simulink model "pv_array"  (Simulink 10.0)
settings: Solver=ode45  StartTime=0.0  StopTime=1.0  RelTol=1e-3  EnableMultiTasking=on
libraries: simulink x8
settings Model: Creator=motahhir  LastModifiedBy=bhisma
settings DataIOCC: LimitDataPoints=on  SignalLoggingSaveFormat=ModelDataLogs
settings OptimizationCC: ExpressionDepthLimit=2147483647
settings DebuggingCC: SolverPrmCheckMsg=warning  FcnCallInpInsideContextMsg=warning  StateNameClashWarn=warning  SFExecutionAtInitializationDiag=warning
settings GRTTargetCC: GeneratePreprocessorConditionals=Disable all  CombineOutputUpdateFcns=on  GRTInterface=off
settings ConfigComp: CovExternalEMLEnable=off  CovSFcnEnable=off

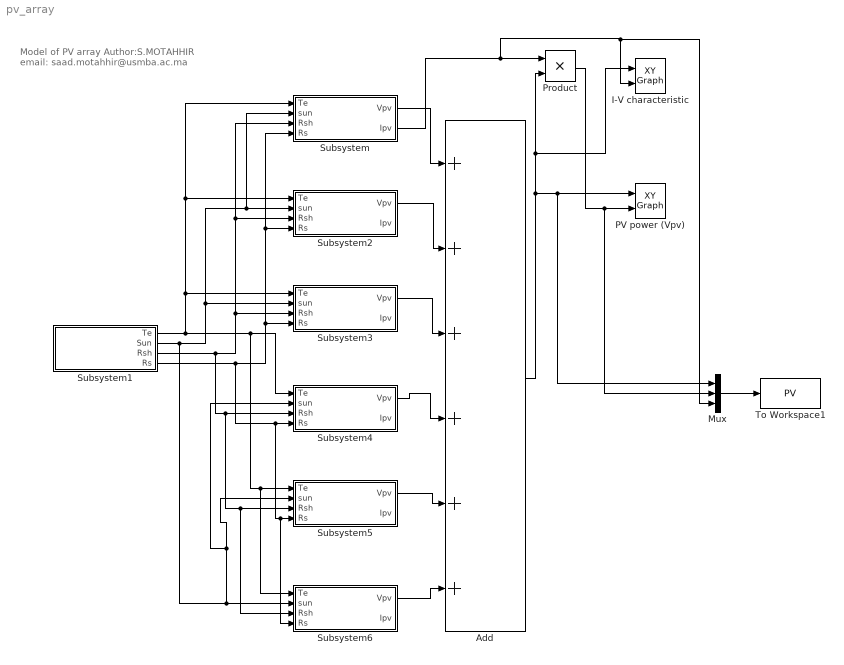
== system pv_array ==
  note: Model of PV array
      | Author:S.MOTAHHIR
      | email: saad.motahhir@usmba.ac.ma
  Add : Sum  Inputs=++++++
  I-V characteristic : simulink/Sinks/XY Graph  xmin=0  xmax=130  ymin=0  ymax=4  st=-1
  Mux : Mux  Inputs=3
  PV power (Vpv) : simulink/Sinks/XY Graph  xmin=0  xmax=130  ymin=0  ymax=400  st=-1
  Product : Product  RndMeth=Zero
  Subsystem : Subsystem
      mask Display:
      | plot([0.3 0.4],[0.4 0.8]);
      | plot([0.4 0.5],[0.4 0.8]);
      | plot([0.5 0.6],[0.4 0.8]);
      | plot([0.6 0.7],[0.4 0.8]);
      | plot([0.3 0.6],[0.4 0.4]);
      | plot([0.325 0.625],[0.5 0.5]);
      | plot([0.35 0.65],[0.6 0.6]);
      | plot([0.375 0.675],[0.7 0.7]);
      | plot([0.4 0.7],[0.8 0.8]);
      | text(0.5,0.9,'PV module (V)','horizontalAlignment', 'center');
  Subsystem1 : Subsystem
  Subsystem2 : Subsystem
      mask Display:
      | plot([0.3 0.4],[0.4 0.8]);
      | plot([0.4 0.5],[0.4 0.8]);
      | plot([0.5 0.6],[0.4 0.8]);
      | plot([0.6 0.7],[0.4 0.8]);
      | plot([0.3 0.6],[0.4 0.4]);
      | plot([0.325 0.625],[0.5 0.5]);
      | plot([0.35 0.65],[0.6 0.6]);
      | plot([0.375 0.675],[0.7 0.7]);
      | plot([0.4 0.7],[0.8 0.8]);
      | text(0.5,0.9,'PV module (V)','horizontalAlignment', 'center');
  Subsystem3 : Subsystem
      mask Display:
      | plot([0.3 0.4],[0.4 0.8]);
      | plot([0.4 0.5],[0.4 0.8]);
      | plot([0.5 0.6],[0.4 0.8]);
      | plot([0.6 0.7],[0.4 0.8]);
      | plot([0.3 0.6],[0.4 0.4]);
      | plot([0.325 0.625],[0.5 0.5]);
      | plot([0.35 0.65],[0.6 0.6]);
      | plot([0.375 0.675],[0.7 0.7]);
      | plot([0.4 0.7],[0.8 0.8]);
      | text(0.5,0.9,'PV module (V)','horizontalAlignment', 'center');
  Subsystem4 : Subsystem
      mask Display:
      | plot([0.3 0.4],[0.4 0.8]);
      | plot([0.4 0.5],[0.4 0.8]);
      | plot([0.5 0.6],[0.4 0.8]);
      | plot([0.6 0.7],[0.4 0.8]);
      | plot([0.3 0.6],[0.4 0.4]);
      | plot([0.325 0.625],[0.5 0.5]);
      | plot([0.35 0.65],[0.6 0.6]);
      | plot([0.375 0.675],[0.7 0.7]);
      | plot([0.4 0.7],[0.8 0.8]);
      | text(0.5,0.9,'PV module (V)','horizontalAlignment', 'center');
  Subsystem5 : Subsystem
      mask Display:
      | plot([0.3 0.4],[0.4 0.8]);
      | plot([0.4 0.5],[0.4 0.8]);
      | plot([0.5 0.6],[0.4 0.8]);
      | plot([0.6 0.7],[0.4 0.8]);
      | plot([0.3 0.6],[0.4 0.4]);
      | plot([0.325 0.625],[0.5 0.5]);
      | plot([0.35 0.65],[0.6 0.6]);
      | plot([0.375 0.675],[0.7 0.7]);
      | plot([0.4 0.7],[0.8 0.8]);
      | text(0.5,0.9,'PV module (V)','horizontalAlignment', 'center');
  Subsystem6 : Subsystem
      mask Display:
      | plot([0.3 0.4],[0.4 0.8]);
      | plot([0.4 0.5],[0.4 0.8]);
      | plot([0.5 0.6],[0.4 0.8]);
      | plot([0.6 0.7],[0.4 0.8]);
      | plot([0.3 0.6],[0.4 0.4]);
      | plot([0.325 0.625],[0.5 0.5]);
      | plot([0.35 0.65],[0.6 0.6]);
      | plot([0.375 0.675],[0.7 0.7]);
      | plot([0.4 0.7],[0.8 0.8]);
      | text(0.5,0.9,'PV module (V)','horizontalAlignment', 'center');
  To Workspace1 : ToWorkspace  VariableName=PV  SaveFormat=Structure With Time  SampleTime=-1
  wires:
  Subsystem1/1(Te) -> Subsystem3/1(Te), Subsystem2/1(Te), Subsystem/1(Te), Subsystem4/1(Te), Subsystem6/1(Te), Subsystem5/1(Te)
  Subsystem1/3(Rsh) -> Subsystem3/3(Rsh), Subsystem2/3(Rsh), Subsystem/3(Rsh), Subsystem4/3(Rsh), Subsystem6/3(Rsh), Subsystem5/3(Rsh)
  Subsystem1/4(Rs) -> Subsystem3/4(Rs), Subsystem2/4(Rs), Subsystem/4(Rs), Subsystem4/4(Rs), Subsystem6/4(Rs), Subsystem5/4(Rs)
  Subsystem/1(Vpv) -> Add/1
  Subsystem2/1(Vpv) -> Add/2
  Subsystem3/1(Vpv) -> Add/3
  Subsystem4/1(Vpv) -> Add/4
  Subsystem5/1(Vpv) -> Add/5
  Subsystem6/1(Vpv) -> Add/6
  Product/1 -> Mux/2, PV power (Vpv)/2
  Mux/1 -> To Workspace1/1
  Add/1 -> Product/2, I-V characteristic/1, Mux/1, PV power (Vpv)/1
  Subsystem/2(Ipv) -> Product/1, Mux/3, I-V characteristic/2
  Subsystem1/2(Sun) -> Subsystem4/2(sun), Subsystem5/2(sun), Subsystem6/2(sun), Subsystem3/2(sun), Subsystem/2(sun), Subsystem2/2(sun)

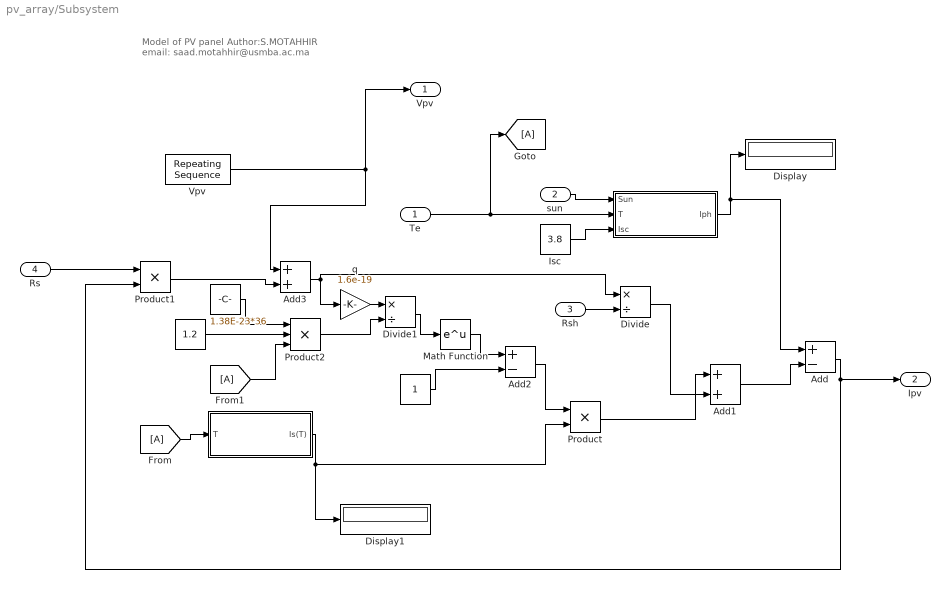
== system pv_array/Subsystem ==
  note: Model of PV panel
      | Author:S.MOTAHHIR
      | email: saad.motahhir@usmba.ac.ma
  Te : Inport
  sun : Inport  Port=2
  Rsh : Inport  Port=3
  Rs : Inport  Port=4
  "  " : Subsystem
  "   " : Subsystem
      mask init:
      | q=1.6e-19;
      | T=298.15;
      | Tnom=298.15;
      | K=1,3806505e-23;
      | N=1.5;
      | vt=36*T*K/q;
      | Is=2.16e-8;
      | Eg=1.12;
  "           " : Constant
  "              " : Constant  Value=1.2
  "               " : Constant  Value=1.38E-23*36
  Add : Sum  Inputs=+-
  Add1 : Sum
  Add2 : Sum  Inputs=+-
  Add3 : Sum
  Display : Display
  Display1 : Display
  Divide : Product  Inputs=*/
  Divide1 : Product  Inputs=*/
  Isc : Constant  Value=3.8
  Math Function : Math  SaturateOnIntegerOverflow=on
  Product : Product  RndMeth=Zero
  Product1 : Product  RndMeth=Zero
  Product2 : Product  Inputs=3  RndMeth=Zero
  "Vpv      " : simulink/Sources/Repeating Sequence  rep_seq_t=[0 1 2]  rep_seq_y="[-0.1  21.5 -0.1]"
  q : Gain  Gain=1.6e-19
  Vpv : Outport
  Ipv : Outport  Port=2
  wires:
  Isc/1 -> "  "/3(Isc)
  Te/1 -> "  "/2(T), [A]
  "  "/1(Iph) -> Display/1, Add/1
  [A] -> "   "/1(T)
  Divide/1 -> Add1/2
  "   "/1(Is(T)) -> Product/2, Display1/1
  Add2/1 -> Product/1
  Math Function/1 -> Add2/1
  "           "/1 -> Add2/2
  Divide1/1 -> Math Function/1
  Product/1 -> Add1/1
  Add1/1 -> Add/2
  q/1 -> Divide1/1
  Add3/1 -> q/1, Divide/1
  "               "/1 -> Product2/1
  [A] -> Product2/3
  "              "/1 -> Product2/2
  Product2/1 -> Divide1/2
  sun/1 -> "  "/1(Sun)
  Rsh/1 -> Divide/2
  Add/1 -> Product1/2, Ipv/1
  Rs/1 -> Product1/1
  Product1/1 -> Add3/2
  "Vpv      "/1 -> Vpv/1, Add3/1

== system pv_array/Subsystem1 ==
  Constant : Constant  Value=298.15
  Constant1 : Constant  Value=1000
  Constant2 : Constant  Value=1000*6
  Constant3 : Constant  Value=0.008*6
  Te : Outport
  Sun : Outport  Port=2
  Rsh : Outport  Port=3
  Rs : Outport  Port=4
  wires:
  Constant/1 -> Te/1
  Constant1/1 -> Sun/1
  Constant3/1 -> Rs/1
  Constant2/1 -> Rsh/1

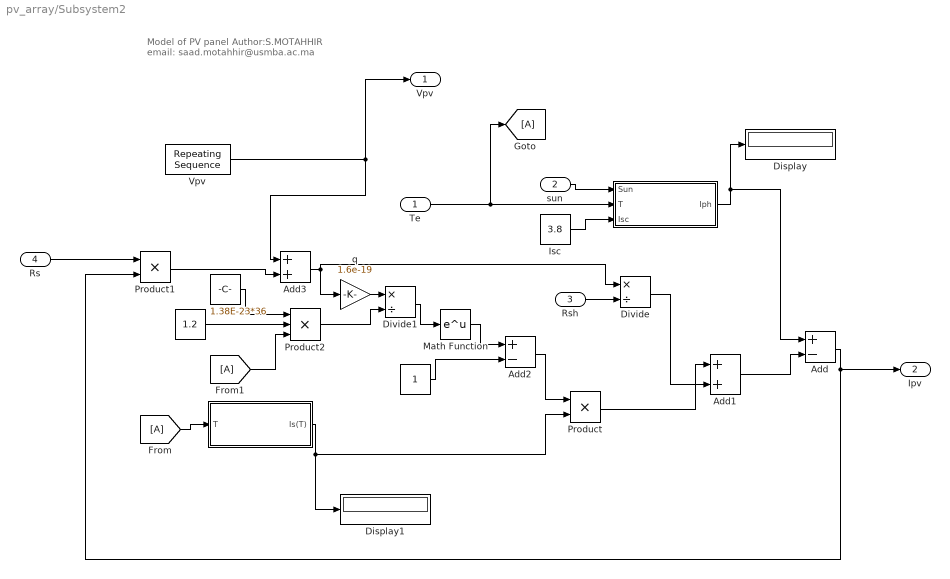
== system pv_array/Subsystem2 ==
  note: Model of PV panel
      | Author:S.MOTAHHIR
      | email: saad.motahhir@usmba.ac.ma
  Te : Inport
  sun : Inport  Port=2
  Rsh : Inport  Port=3
  Rs : Inport  Port=4
  "  " : Subsystem
  "   " : Subsystem
      mask init:
      | q=1.6e-19;
      | T=298.15;
      | Tnom=298.15;
      | K=1,3806505e-23;
      | N=1.5;
      | vt=36*T*K/q;
      | Is=2.16e-8;
      | Eg=1.12;
  "           " : Constant
  "              " : Constant  Value=1.2
  "               " : Constant  Value=1.38E-23*36
  Add : Sum  Inputs=+-
  Add1 : Sum
  Add2 : Sum  Inputs=+-
  Add3 : Sum
  Display : Display
  Display1 : Display
  Divide : Product  Inputs=*/
  Divide1 : Product  Inputs=*/
  Isc : Constant  Value=3.8
  Math Function : Math  SaturateOnIntegerOverflow=on
  Product : Product  RndMeth=Zero
  Product1 : Product  RndMeth=Zero
  Product2 : Product  Inputs=3  RndMeth=Zero
  "Vpv      " : simulink/Sources/Repeating Sequence  rep_seq_t=[0 1 2]  rep_seq_y="[-0.1  21.5 -0.1]"
  q : Gain  Gain=1.6e-19
  Vpv : Outport
  Ipv : Outport  Port=2
  wires:
  Isc/1 -> "  "/3(Isc)
  Te/1 -> "  "/2(T), [A]
  "  "/1(Iph) -> Display/1, Add/1
  [A] -> "   "/1(T)
  Divide/1 -> Add1/2
  "   "/1(Is(T)) -> Product/2, Display1/1
  Add2/1 -> Product/1
  Math Function/1 -> Add2/1
  "           "/1 -> Add2/2
  Divide1/1 -> Math Function/1
  Product/1 -> Add1/1
  Add1/1 -> Add/2
  q/1 -> Divide1/1
  Add3/1 -> q/1, Divide/1
  "               "/1 -> Product2/1
  [A] -> Product2/3
  "              "/1 -> Product2/2
  Product2/1 -> Divide1/2
  sun/1 -> "  "/1(Sun)
  Rsh/1 -> Divide/2
  Add/1 -> Product1/2, Ipv/1
  Rs/1 -> Product1/1
  Product1/1 -> Add3/2
  "Vpv      "/1 -> Vpv/1, Add3/1

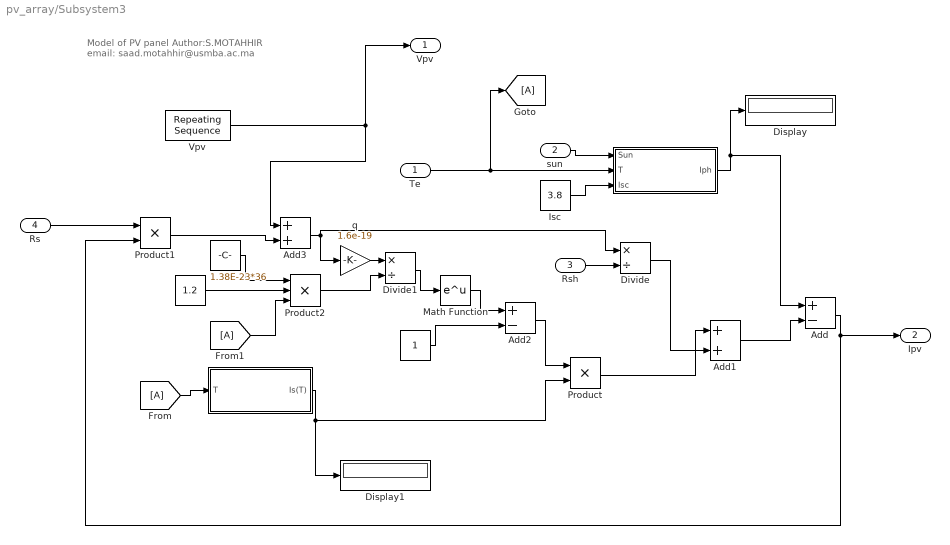
== system pv_array/Subsystem3 ==
  note: Model of PV panel
      | Author:S.MOTAHHIR
      | email: saad.motahhir@usmba.ac.ma
  Te : Inport
  sun : Inport  Port=2
  Rsh : Inport  Port=3
  Rs : Inport  Port=4
  "  " : Subsystem
  "   " : Subsystem
      mask init:
      | q=1.6e-19;
      | T=298.15;
      | Tnom=298.15;
      | K=1,3806505e-23;
      | N=1.5;
      | vt=36*T*K/q;
      | Is=2.16e-8;
      | Eg=1.12;
  "           " : Constant
  "              " : Constant  Value=1.2
  "               " : Constant  Value=1.38E-23*36
  Add : Sum  Inputs=+-
  Add1 : Sum
  Add2 : Sum  Inputs=+-
  Add3 : Sum
  Display : Display
  Display1 : Display
  Divide : Product  Inputs=*/
  Divide1 : Product  Inputs=*/
  Isc : Constant  Value=3.8
  Math Function : Math  SaturateOnIntegerOverflow=on
  Product : Product  RndMeth=Zero
  Product1 : Product  RndMeth=Zero
  Product2 : Product  Inputs=3  RndMeth=Zero
  "Vpv      " : simulink/Sources/Repeating Sequence  rep_seq_t=[0 1 2]  rep_seq_y="[-0.1  21.5 -0.1]"
  q : Gain  Gain=1.6e-19
  Vpv : Outport
  Ipv : Outport  Port=2
  wires:
  Isc/1 -> "  "/3(Isc)
  Te/1 -> "  "/2(T), [A]
  "  "/1(Iph) -> Display/1, Add/1
  [A] -> "   "/1(T)
  Divide/1 -> Add1/2
  "   "/1(Is(T)) -> Product/2, Display1/1
  Add2/1 -> Product/1
  Math Function/1 -> Add2/1
  "           "/1 -> Add2/2
  Divide1/1 -> Math Function/1
  Product/1 -> Add1/1
  Add1/1 -> Add/2
  q/1 -> Divide1/1
  Add3/1 -> q/1, Divide/1
  "               "/1 -> Product2/1
  [A] -> Product2/3
  "              "/1 -> Product2/2
  Product2/1 -> Divide1/2
  sun/1 -> "  "/1(Sun)
  Rsh/1 -> Divide/2
  Add/1 -> Product1/2, Ipv/1
  Rs/1 -> Product1/1
  Product1/1 -> Add3/2
  "Vpv      "/1 -> Vpv/1, Add3/1

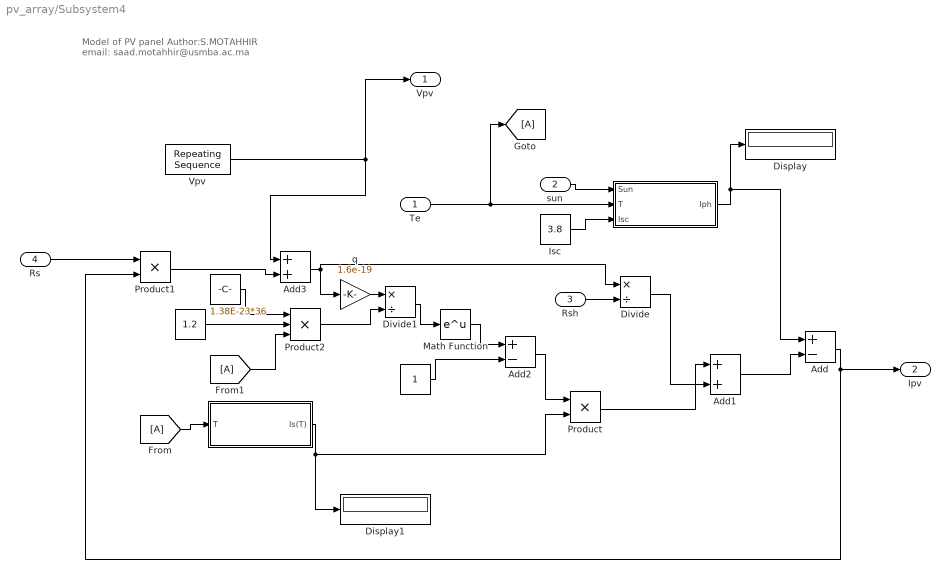
== system pv_array/Subsystem4 ==
  note: Model of PV panel
      | Author:S.MOTAHHIR
      | email: saad.motahhir@usmba.ac.ma
  Te : Inport
  sun : Inport  Port=2
  Rsh : Inport  Port=3
  Rs : Inport  Port=4
  "  " : Subsystem
  "   " : Subsystem
      mask init:
      | q=1.6e-19;
      | T=298.15;
      | Tnom=298.15;
      | K=1,3806505e-23;
      | N=1.5;
      | vt=36*T*K/q;
      | Is=2.16e-8;
      | Eg=1.12;
  "           " : Constant
  "              " : Constant  Value=1.2
  "               " : Constant  Value=1.38E-23*36
  Add : Sum  Inputs=+-
  Add1 : Sum
  Add2 : Sum  Inputs=+-
  Add3 : Sum
  Display : Display
  Display1 : Display
  Divide : Product  Inputs=*/
  Divide1 : Product  Inputs=*/
  Isc : Constant  Value=3.8
  Math Function : Math  SaturateOnIntegerOverflow=on
  Product : Product  RndMeth=Zero
  Product1 : Product  RndMeth=Zero
  Product2 : Product  Inputs=3  RndMeth=Zero
  "Vpv      " : simulink/Sources/Repeating Sequence  rep_seq_t=[0 1 2]  rep_seq_y="[-0.1  21.5 -0.1]"
  q : Gain  Gain=1.6e-19
  Vpv : Outport
  Ipv : Outport  Port=2
  wires:
  Isc/1 -> "  "/3(Isc)
  Te/1 -> "  "/2(T), [A]
  "  "/1(Iph) -> Display/1, Add/1
  [A] -> "   "/1(T)
  Divide/1 -> Add1/2
  "   "/1(Is(T)) -> Product/2, Display1/1
  Add2/1 -> Product/1
  Math Function/1 -> Add2/1
  "           "/1 -> Add2/2
  Divide1/1 -> Math Function/1
  Product/1 -> Add1/1
  Add1/1 -> Add/2
  q/1 -> Divide1/1
  Add3/1 -> q/1, Divide/1
  "               "/1 -> Product2/1
  [A] -> Product2/3
  "              "/1 -> Product2/2
  Product2/1 -> Divide1/2
  sun/1 -> "  "/1(Sun)
  Rsh/1 -> Divide/2
  Add/1 -> Product1/2, Ipv/1
  Rs/1 -> Product1/1
  Product1/1 -> Add3/2
  "Vpv      "/1 -> Vpv/1, Add3/1

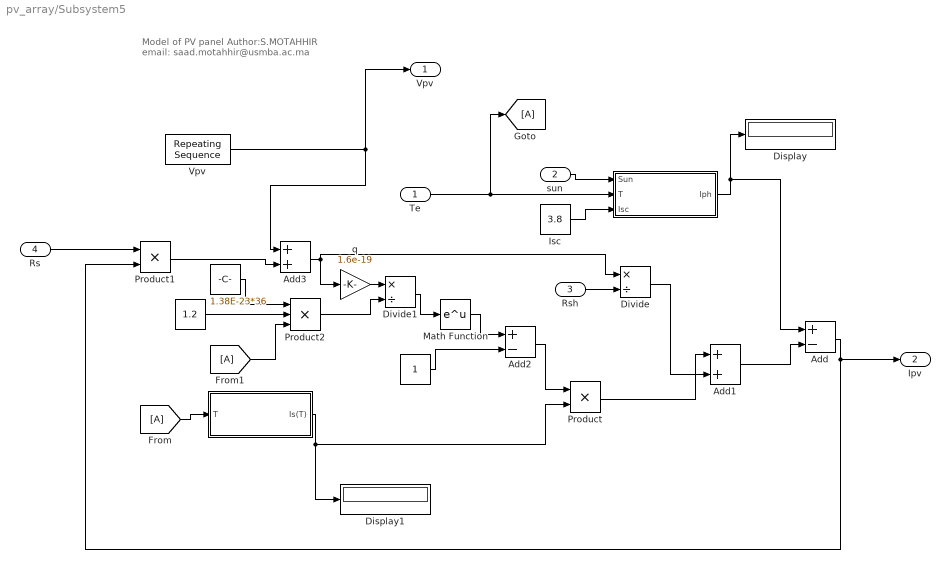
== system pv_array/Subsystem5 ==
  note: Model of PV panel
      | Author:S.MOTAHHIR
      | email: saad.motahhir@usmba.ac.ma
  Te : Inport
  sun : Inport  Port=2
  Rsh : Inport  Port=3
  Rs : Inport  Port=4
  "  " : Subsystem
  "   " : Subsystem
      mask init:
      | q=1.6e-19;
      | T=298.15;
      | Tnom=298.15;
      | K=1,3806505e-23;
      | N=1.5;
      | vt=36*T*K/q;
      | Is=2.16e-8;
      | Eg=1.12;
  "           " : Constant
  "              " : Constant  Value=1.2
  "               " : Constant  Value=1.38E-23*36
  Add : Sum  Inputs=+-
  Add1 : Sum
  Add2 : Sum  Inputs=+-
  Add3 : Sum
  Display : Display
  Display1 : Display
  Divide : Product  Inputs=*/
  Divide1 : Product  Inputs=*/
  Isc : Constant  Value=3.8
  Math Function : Math  SaturateOnIntegerOverflow=on
  Product : Product  RndMeth=Zero
  Product1 : Product  RndMeth=Zero
  Product2 : Product  Inputs=3  RndMeth=Zero
  "Vpv      " : simulink/Sources/Repeating Sequence  rep_seq_t=[0 1 2]  rep_seq_y="[-0.1  21.5 -0.1]"
  q : Gain  Gain=1.6e-19
  Vpv : Outport
  Ipv : Outport  Port=2
  wires:
  Isc/1 -> "  "/3(Isc)
  Te/1 -> "  "/2(T), [A]
  "  "/1(Iph) -> Display/1, Add/1
  [A] -> "   "/1(T)
  Divide/1 -> Add1/2
  "   "/1(Is(T)) -> Product/2, Display1/1
  Add2/1 -> Product/1
  Math Function/1 -> Add2/1
  "           "/1 -> Add2/2
  Divide1/1 -> Math Function/1
  Product/1 -> Add1/1
  Add1/1 -> Add/2
  q/1 -> Divide1/1
  Add3/1 -> q/1, Divide/1
  "               "/1 -> Product2/1
  [A] -> Product2/3
  "              "/1 -> Product2/2
  Product2/1 -> Divide1/2
  sun/1 -> "  "/1(Sun)
  Rsh/1 -> Divide/2
  Add/1 -> Product1/2, Ipv/1
  Rs/1 -> Product1/1
  Product1/1 -> Add3/2
  "Vpv      "/1 -> Vpv/1, Add3/1

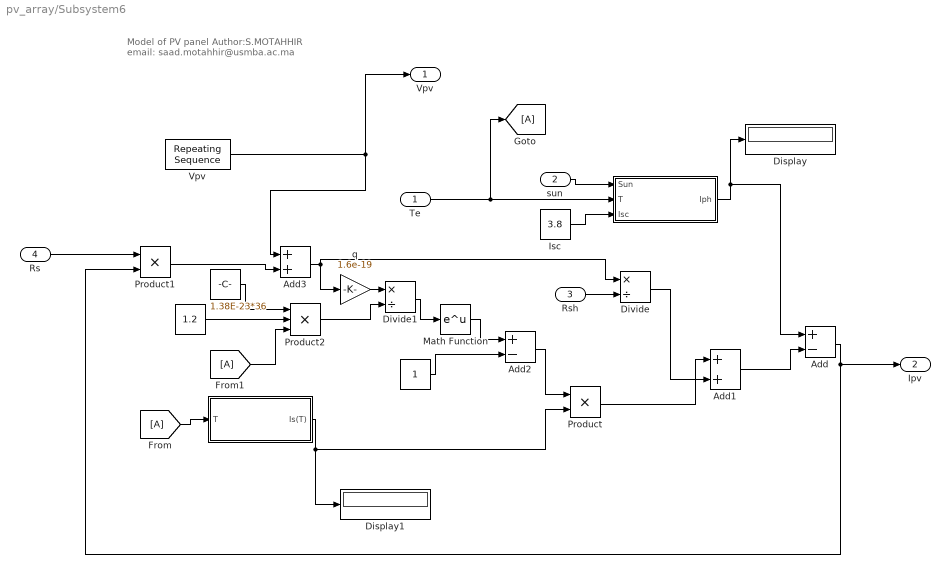
== system pv_array/Subsystem6 ==
  note: Model of PV panel
      | Author:S.MOTAHHIR
      | email: saad.motahhir@usmba.ac.ma
  Te : Inport
  sun : Inport  Port=2
  Rsh : Inport  Port=3
  Rs : Inport  Port=4
  "  " : Subsystem
  "   " : Subsystem
      mask init:
      | q=1.6e-19;
      | T=298.15;
      | Tnom=298.15;
      | K=1,3806505e-23;
      | N=1.5;
      | vt=36*T*K/q;
      | Is=2.16e-8;
      | Eg=1.12;
  "           " : Constant
  "              " : Constant  Value=1.2
  "               " : Constant  Value=1.38E-23*36
  Add : Sum  Inputs=+-
  Add1 : Sum
  Add2 : Sum  Inputs=+-
  Add3 : Sum
  Display : Display
  Display1 : Display
  Divide : Product  Inputs=*/
  Divide1 : Product  Inputs=*/
  Isc : Constant  Value=3.8
  Math Function : Math  SaturateOnIntegerOverflow=on
  Product : Product  RndMeth=Zero
  Product1 : Product  RndMeth=Zero
  Product2 : Product  Inputs=3  RndMeth=Zero
  "Vpv      " : simulink/Sources/Repeating Sequence  rep_seq_t=[0 1 2]  rep_seq_y="[-0.1  21.5 -0.1]"
  q : Gain  Gain=1.6e-19
  Vpv : Outport
  Ipv : Outport  Port=2
  wires:
  Isc/1 -> "  "/3(Isc)
  Te/1 -> "  "/2(T), [A]
  "  "/1(Iph) -> Display/1, Add/1
  [A] -> "   "/1(T)
  Divide/1 -> Add1/2
  "   "/1(Is(T)) -> Product/2, Display1/1
  Add2/1 -> Product/1
  Math Function/1 -> Add2/1
  "           "/1 -> Add2/2
  Divide1/1 -> Math Function/1
  Product/1 -> Add1/1
  Add1/1 -> Add/2
  q/1 -> Divide1/1
  Add3/1 -> q/1, Divide/1
  "               "/1 -> Product2/1
  [A] -> Product2/3
  "              "/1 -> Product2/2
  Product2/1 -> Divide1/2
  sun/1 -> "  "/1(Sun)
  Rsh/1 -> Divide/2
  Add/1 -> Product1/2, Ipv/1
  Rs/1 -> Product1/1
  Product1/1 -> Add3/2
  "Vpv      "/1 -> Vpv/1, Add3/1

== system pv_array/Subsystem/   ==
  Sun : Inport
  T : Inport  Port=2
  Isc : Inport  Port=3
  "   " : Constant  Value=0.0017
  "    " : Constant  Value=1000
  "      " : Constant  Value=298
  Add : Sum  Inputs=+-
  Add1 : Sum
  Divide : Product  Inputs=*/
  Product : Product  RndMeth=Zero
  Product1 : Product  RndMeth=Zero
  Iph : Outport
  wires:
  Product/1 -> Iph/1
  Sun/1 -> Divide/1
  "    "/1 -> Divide/2
  T/1 -> Add/1
  "      "/1 -> Add/2
  Add/1 -> Product1/1
  "   "/1 -> Product1/2
  Product1/1 -> Add1/1
  Add1/1 -> Product/2
  Isc/1 -> Add1/2
  Divide/1 -> Product/1

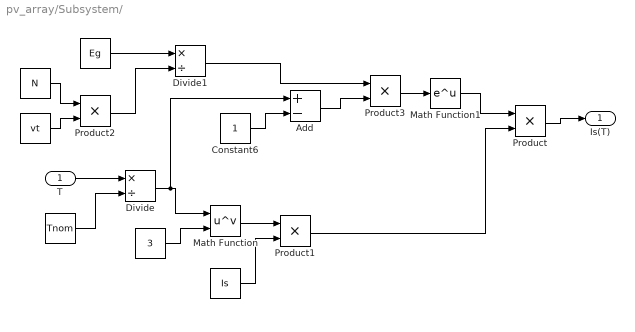
== system pv_array/Subsystem/    ==
  T : Inport
  "  " : Constant  Value=3
  "      " : Constant  Value=Is
  "        " : Constant  Value=Tnom
  "                      " : Constant  Value=Eg
  "                              " : Constant  Value=N
  "                               " : Constant  Value=vt
  Add : Sum  Inputs=+-
  Constant6 : Constant
  Divide : Product  Inputs=*/
  Divide1 : Product  Inputs=*/
  Math Function : Math  Operator=pow  SaturateOnIntegerOverflow=on
  Math Function1 : Math  SaturateOnIntegerOverflow=on
  Product{,1..3} (4 alike) : Product  RndMeth=Zero
  Is(T) : Outport
  wires:
  Product/1 -> Is(T)/1
  T/1 -> Divide/1
  "        "/1 -> Divide/2
  Divide/1 -> Math Function/1, Add/1
  "  "/1 -> Math Function/2
  Math Function/1 -> Product1/1
  "      "/1 -> Product1/2
  Product1/1 -> Product/2
  "                               "/1 -> Product2/2
  "                              "/1 -> Product2/1
  Product2/1 -> Divide1/2
  "                      "/1 -> Divide1/1
  Math Function1/1 -> Product/1
  Product3/1 -> Math Function1/1
  Divide1/1 -> Product3/1
  Add/1 -> Product3/2
  Constant6/1 -> Add/2

== system pv_array/Subsystem2/   ==
  Sun : Inport
  T : Inport  Port=2
  Isc : Inport  Port=3
  "   " : Constant  Value=0.0017
  "    " : Constant  Value=1000
  "      " : Constant  Value=298
  Add : Sum  Inputs=+-
  Add1 : Sum
  Divide : Product  Inputs=*/
  Product : Product  RndMeth=Zero
  Product1 : Product  RndMeth=Zero
  Iph : Outport
  wires:
  Product/1 -> Iph/1
  Sun/1 -> Divide/1
  "    "/1 -> Divide/2
  T/1 -> Add/1
  "      "/1 -> Add/2
  Add/1 -> Product1/1
  "   "/1 -> Product1/2
  Product1/1 -> Add1/1
  Add1/1 -> Product/2
  Isc/1 -> Add1/2
  Divide/1 -> Product/1

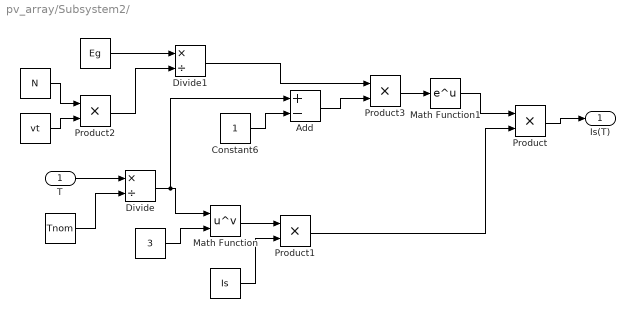
== system pv_array/Subsystem2/    ==
  T : Inport
  "  " : Constant  Value=3
  "      " : Constant  Value=Is
  "        " : Constant  Value=Tnom
  "                      " : Constant  Value=Eg
  "                              " : Constant  Value=N
  "                               " : Constant  Value=vt
  Add : Sum  Inputs=+-
  Constant6 : Constant
  Divide : Product  Inputs=*/
  Divide1 : Product  Inputs=*/
  Math Function : Math  Operator=pow  SaturateOnIntegerOverflow=on
  Math Function1 : Math  SaturateOnIntegerOverflow=on
  Product{,1..3} (4 alike) : Product  RndMeth=Zero
  Is(T) : Outport
  wires:
  Product/1 -> Is(T)/1
  T/1 -> Divide/1
  "        "/1 -> Divide/2
  Divide/1 -> Math Function/1, Add/1
  "  "/1 -> Math Function/2
  Math Function/1 -> Product1/1
  "      "/1 -> Product1/2
  Product1/1 -> Product/2
  "                               "/1 -> Product2/2
  "                              "/1 -> Product2/1
  Product2/1 -> Divide1/2
  "                      "/1 -> Divide1/1
  Math Function1/1 -> Product/1
  Product3/1 -> Math Function1/1
  Divide1/1 -> Product3/1
  Add/1 -> Product3/2
  Constant6/1 -> Add/2

== system pv_array/Subsystem3/   ==
  Sun : Inport
  T : Inport  Port=2
  Isc : Inport  Port=3
  "   " : Constant  Value=0.0017
  "    " : Constant  Value=1000
  "      " : Constant  Value=298
  Add : Sum  Inputs=+-
  Add1 : Sum
  Divide : Product  Inputs=*/
  Product : Product  RndMeth=Zero
  Product1 : Product  RndMeth=Zero
  Iph : Outport
  wires:
  Product/1 -> Iph/1
  Sun/1 -> Divide/1
  "    "/1 -> Divide/2
  T/1 -> Add/1
  "      "/1 -> Add/2
  Add/1 -> Product1/1
  "   "/1 -> Product1/2
  Product1/1 -> Add1/1
  Add1/1 -> Product/2
  Isc/1 -> Add1/2
  Divide/1 -> Product/1

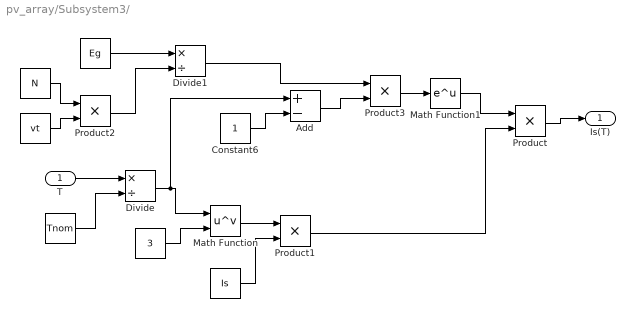
== system pv_array/Subsystem3/    ==
  T : Inport
  "  " : Constant  Value=3
  "      " : Constant  Value=Is
  "        " : Constant  Value=Tnom
  "                      " : Constant  Value=Eg
  "                              " : Constant  Value=N
  "                               " : Constant  Value=vt
  Add : Sum  Inputs=+-
  Constant6 : Constant
  Divide : Product  Inputs=*/
  Divide1 : Product  Inputs=*/
  Math Function : Math  Operator=pow  SaturateOnIntegerOverflow=on
  Math Function1 : Math  SaturateOnIntegerOverflow=on
  Product{,1..3} (4 alike) : Product  RndMeth=Zero
  Is(T) : Outport
  wires:
  Product/1 -> Is(T)/1
  T/1 -> Divide/1
  "        "/1 -> Divide/2
  Divide/1 -> Math Function/1, Add/1
  "  "/1 -> Math Function/2
  Math Function/1 -> Product1/1
  "      "/1 -> Product1/2
  Product1/1 -> Product/2
  "                               "/1 -> Product2/2
  "                              "/1 -> Product2/1
  Product2/1 -> Divide1/2
  "                      "/1 -> Divide1/1
  Math Function1/1 -> Product/1
  Product3/1 -> Math Function1/1
  Divide1/1 -> Product3/1
  Add/1 -> Product3/2
  Constant6/1 -> Add/2

== system pv_array/Subsystem4/   ==
  Sun : Inport
  T : Inport  Port=2
  Isc : Inport  Port=3
  "   " : Constant  Value=0.0017
  "    " : Constant  Value=1000
  "      " : Constant  Value=298
  Add : Sum  Inputs=+-
  Add1 : Sum
  Divide : Product  Inputs=*/
  Product : Product  RndMeth=Zero
  Product1 : Product  RndMeth=Zero
  Iph : Outport
  wires:
  Product/1 -> Iph/1
  Sun/1 -> Divide/1
  "    "/1 -> Divide/2
  T/1 -> Add/1
  "      "/1 -> Add/2
  Add/1 -> Product1/1
  "   "/1 -> Product1/2
  Product1/1 -> Add1/1
  Add1/1 -> Product/2
  Isc/1 -> Add1/2
  Divide/1 -> Product/1

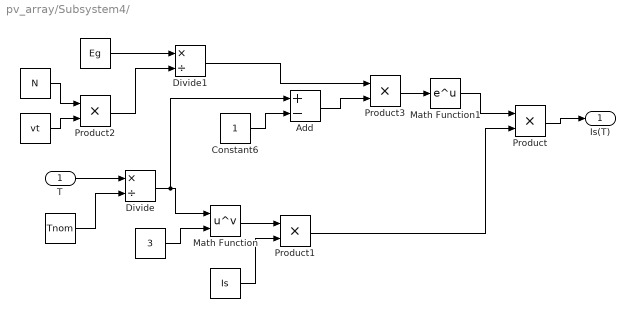
== system pv_array/Subsystem4/    ==
  T : Inport
  "  " : Constant  Value=3
  "      " : Constant  Value=Is
  "        " : Constant  Value=Tnom
  "                      " : Constant  Value=Eg
  "                              " : Constant  Value=N
  "                               " : Constant  Value=vt
  Add : Sum  Inputs=+-
  Constant6 : Constant
  Divide : Product  Inputs=*/
  Divide1 : Product  Inputs=*/
  Math Function : Math  Operator=pow  SaturateOnIntegerOverflow=on
  Math Function1 : Math  SaturateOnIntegerOverflow=on
  Product{,1..3} (4 alike) : Product  RndMeth=Zero
  Is(T) : Outport
  wires:
  Product/1 -> Is(T)/1
  T/1 -> Divide/1
  "        "/1 -> Divide/2
  Divide/1 -> Math Function/1, Add/1
  "  "/1 -> Math Function/2
  Math Function/1 -> Product1/1
  "      "/1 -> Product1/2
  Product1/1 -> Product/2
  "                               "/1 -> Product2/2
  "                              "/1 -> Product2/1
  Product2/1 -> Divide1/2
  "                      "/1 -> Divide1/1
  Math Function1/1 -> Product/1
  Product3/1 -> Math Function1/1
  Divide1/1 -> Product3/1
  Add/1 -> Product3/2
  Constant6/1 -> Add/2

== system pv_array/Subsystem5/   ==
  Sun : Inport
  T : Inport  Port=2
  Isc : Inport  Port=3
  "   " : Constant  Value=0.0017
  "    " : Constant  Value=1000
  "      " : Constant  Value=298
  Add : Sum  Inputs=+-
  Add1 : Sum
  Divide : Product  Inputs=*/
  Product : Product  RndMeth=Zero
  Product1 : Product  RndMeth=Zero
  Iph : Outport
  wires:
  Product/1 -> Iph/1
  Sun/1 -> Divide/1
  "    "/1 -> Divide/2
  T/1 -> Add/1
  "      "/1 -> Add/2
  Add/1 -> Product1/1
  "   "/1 -> Product1/2
  Product1/1 -> Add1/1
  Add1/1 -> Product/2
  Isc/1 -> Add1/2
  Divide/1 -> Product/1

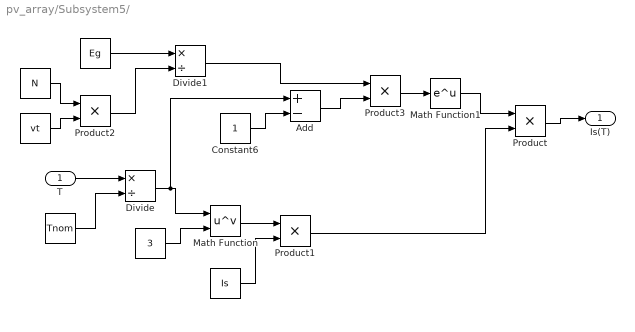
== system pv_array/Subsystem5/    ==
  T : Inport
  "  " : Constant  Value=3
  "      " : Constant  Value=Is
  "        " : Constant  Value=Tnom
  "                      " : Constant  Value=Eg
  "                              " : Constant  Value=N
  "                               " : Constant  Value=vt
  Add : Sum  Inputs=+-
  Constant6 : Constant
  Divide : Product  Inputs=*/
  Divide1 : Product  Inputs=*/
  Math Function : Math  Operator=pow  SaturateOnIntegerOverflow=on
  Math Function1 : Math  SaturateOnIntegerOverflow=on
  Product{,1..3} (4 alike) : Product  RndMeth=Zero
  Is(T) : Outport
  wires:
  Product/1 -> Is(T)/1
  T/1 -> Divide/1
  "        "/1 -> Divide/2
  Divide/1 -> Math Function/1, Add/1
  "  "/1 -> Math Function/2
  Math Function/1 -> Product1/1
  "      "/1 -> Product1/2
  Product1/1 -> Product/2
  "                               "/1 -> Product2/2
  "                              "/1 -> Product2/1
  Product2/1 -> Divide1/2
  "                      "/1 -> Divide1/1
  Math Function1/1 -> Product/1
  Product3/1 -> Math Function1/1
  Divide1/1 -> Product3/1
  Add/1 -> Product3/2
  Constant6/1 -> Add/2

== system pv_array/Subsystem6/   ==
  Sun : Inport
  T : Inport  Port=2
  Isc : Inport  Port=3
  "   " : Constant  Value=0.0017
  "    " : Constant  Value=1000
  "      " : Constant  Value=298
  Add : Sum  Inputs=+-
  Add1 : Sum
  Divide : Product  Inputs=*/
  Product : Product  RndMeth=Zero
  Product1 : Product  RndMeth=Zero
  Iph : Outport
  wires:
  Product/1 -> Iph/1
  Sun/1 -> Divide/1
  "    "/1 -> Divide/2
  T/1 -> Add/1
  "      "/1 -> Add/2
  Add/1 -> Product1/1
  "   "/1 -> Product1/2
  Product1/1 -> Add1/1
  Add1/1 -> Product/2
  Isc/1 -> Add1/2
  Divide/1 -> Product/1

== system pv_array/Subsystem6/    ==
  T : Inport
  "  " : Constant  Value=3
  "      " : Constant  Value=Is
  "        " : Constant  Value=Tnom
  "                      " : Constant  Value=Eg
  "                              " : Constant  Value=N
  "                               " : Constant  Value=vt
  Add : Sum  Inputs=+-
  Constant6 : Constant
  Divide : Product  Inputs=*/
  Divide1 : Product  Inputs=*/
  Math Function : Math  Operator=pow  SaturateOnIntegerOverflow=on
  Math Function1 : Math  SaturateOnIntegerOverflow=on
  Product{,1..3} (4 alike) : Product  RndMeth=Zero
  Is(T) : Outport
  wires:
  Product/1 -> Is(T)/1
  T/1 -> Divide/1
  "        "/1 -> Divide/2
  Divide/1 -> Math Function/1, Add/1
  "  "/1 -> Math Function/2
  Math Function/1 -> Product1/1
  "      "/1 -> Product1/2
  Product1/1 -> Product/2
  "                               "/1 -> Product2/2
  "                              "/1 -> Product2/1
  Product2/1 -> Divide1/2
  "                      "/1 -> Divide1/1
  Math Function1/1 -> Product/1
  Product3/1 -> Math Function1/1
  Divide1/1 -> Product3/1
  Add/1 -> Product3/2
  Constant6/1 -> Add/2
